simulink library "RobotControlLib"  (R2016b)
settings: Solver=VariableStepAuto  StartTime=0.0  StopTime=10.0  RelTol=1e-3
values from neighbouring files (symbols this model uses):
  CAL_EAST = int16(0)    [ControlInit.m]
  CAL_hitBackwardDist_mm = single(150)    [ControlInit.m]
  CAL_NORTH = int16(270)    [ControlInit.m]
  CAL_PwmMoveThd_mm = uint8(180)    [ControlInit.m]
  CAL_SOUTH = int16(90)    [ControlInit.m]
  CAL_WEST = int16(180)    [ControlInit.m]
  CONST_Zero = int16(0)    [ControlInit.m]
  ENU_DIAG = uint8(28)    [ControlInit.m]
  ENU_END = uint8(27)    [ControlInit.m]
  ENU_SHIFT_HEADING = uint8(29)    [ControlInit.m]
libraries: COMH x1, DSCA x1, ROTH x1, MOVH x1, SCAN x1, MOTH x1
settings Model: Creator=oelkawok  LastModifiedBy=oelkawok

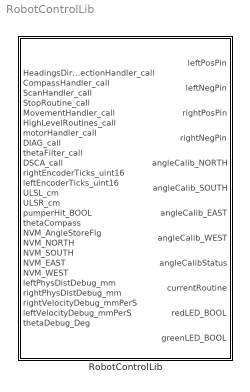
== system RobotControlLib ==
  RobotControlLib : Subsystem

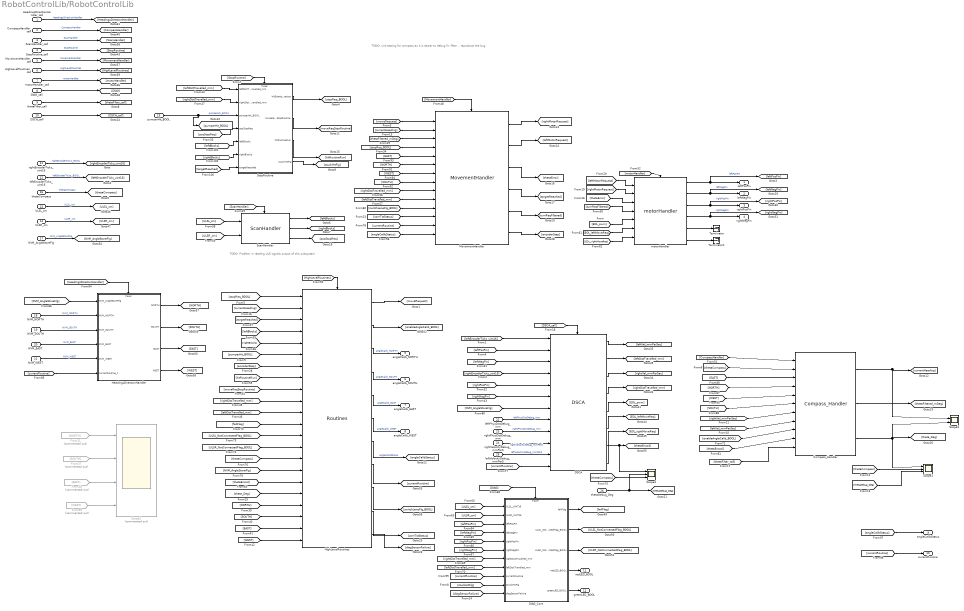
== system RobotControlLib/RobotControlLib ==
  note: TODO: Problem in reading ULS signals output of this subsystem
  note: TODO: unit testing for compass as it is easier to debug fix filter... reproduce the bug
  HeadingsDirectionHandler_call : Inport  PortDimensions=1
  CompassHandler_call : Inport  Port=2  PortDimensions=1
  ScanHandler_call : Inport  Port=3  PortDimensions=1
  StopRoutine_call : Inport  Port=4  PortDimensions=1
  MovementHandler_call : Inport  Port=5  PortDimensions=1
  HighLevelRoutines_call : Inport  Port=6  PortDimensions=1
  motorHandler_call : Inport  Port=7  PortDimensions=1
  DIAG_call : Inport  Port=8  PortDimensions=1
  thetaFilter_call : Inport  Port=9  PortDimensions=1
  DSCA_call : Inport  Port=10  PortDimensions=1
  rightEncoderTicks_uint16 : Inport  Port=11  PortDimensions=1
  leftEncoderTicks_uint16 : Inport  Port=12  PortDimensions=1
  ULSL_cm : Inport  Port=13  PortDimensions=1
  ULSR_cm : Inport  Port=14  PortDimensions=1
  pumperHit_BOOL : Inport  Port=15  OutDataTypeStr=boolean  PortDimensions=1
  thetaCompass : Inport  Port=16  OutDataTypeStr=int16  PortDimensions=1
  NVM_AngleStoreFlg : Inport  Port=17  PortDimensions=1
  NVM_NORTH : Inport  Port=18  PortDimensions=1
  NVM_SOUTH : Inport  Port=19  PortDimensions=1
  NVM_EAST : Inport  Port=20  PortDimensions=1
  NVM_WEST : Inport  Port=21  PortDimensions=1
  leftPhysDistDebug_mm : Inport  Port=22
  rightPhysDistDebug_mm : Inport  Port=23
  rightVelocityDebug_mmPerS : Inport  Port=24
  leftVelocityDebug_mmPerS : Inport  Port=25
  thetaDebug_Deg : Inport  Port=26
  Compass_Handler : COMH/Compass_Handler
  DIAG_Cont : Subsystem
      settings: RTWSystemCode=Nonreusable function  RTWFcnNameOpts=Use subsystem name  RTWFileNameOpts=Use subsystem name  FunctionInterfaceSpec=Allow arguments
  DSCA : DSCA/DSCA
  From21 : From  Commented=on  GotoTag=NORTH
  From37 : From  Commented=on  GotoTag=SOUTH
  From38 : From  Commented=on  GotoTag=EAST
  From95 : From  Commented=on  GotoTag=WEST
  HeadingsDirectionHandler : Subsystem
      settings: RTWSystemCode=Nonreusable function  RTWFcnNameOpts=Use subsystem name  RTWFileNameOpts=Use subsystem name  FunctionInterfaceSpec=Allow arguments
  HighLevelRoutines : ROTH/Routines
  MovementHandler : MOVH/MovementHandler
  ScanHandler : SCAN/ScanHandler
  Scope1 : Scope  NumInputPorts=3
  Scope2 : Scope  Commented=on  NumInputPorts=4
  Scope3 : Scope  NumInputPorts=2
  Scope4 : Scope  NumInputPorts=3
  StopRoutine : Subsystem
      settings: RTWSystemCode=Nonreusable function  RTWFcnNameOpts=Use subsystem name  RTWFileNameOpts=Use subsystem name  FunctionInterfaceSpec=Allow arguments
  Terminator : Terminator
  Terminator1 : Terminator
  motorHandler : MOTH/motorHandler
  leftPosPin : Outport  OutDataTypeStr=uint8  PortDimensions=1
      settings: AttributesFormatString=|
      | Mode: %<OutputWhenDisabled>
      | Init: %<InitialOutput>
  leftNegPin : Outport  Port=2  OutDataTypeStr=uint8  PortDimensions=1
      settings: AttributesFormatString=|
      | Mode: %<OutputWhenDisabled>
      | Init: %<InitialOutput>
  rightPosPin : Outport  Port=3  OutDataTypeStr=uint8  PortDimensions=1
      settings: AttributesFormatString=|
      | Mode: %<OutputWhenDisabled>
      | Init: %<InitialOutput>
  rightNegPin : Outport  Port=4  OutDataTypeStr=uint8  PortDimensions=1
      settings: AttributesFormatString=|
      | Mode: %<OutputWhenDisabled>
      | Init: %<InitialOutput>
  angleCalib_NORTH : Outport  Port=5  InitialOutput=0
      settings: AttributesFormatString=|
      | Mode: %<OutputWhenDisabled>
      | Init: %<InitialOutput>
  angleCalib_SOUTH : Outport  Port=6  InitialOutput=0
      settings: AttributesFormatString=|
      | Mode: %<OutputWhenDisabled>
      | Init: %<InitialOutput>
  angleCalib_EAST : Outport  Port=7  InitialOutput=0
      settings: AttributesFormatString=|
      | Mode: %<OutputWhenDisabled>
      | Init: %<InitialOutput>
  angleCalib_WEST : Outport  Port=8  InitialOutput=0
      settings: AttributesFormatString=|
      | Mode: %<OutputWhenDisabled>
      | Init: %<InitialOutput>
  angleCalibStatus : Outport  Port=9
      settings: AttributesFormatString=|
      | Mode: %<OutputWhenDisabled>
      | Init: %<InitialOutput>
  currentRoutine : Outport  Port=10
      settings: AttributesFormatString=|
      | Mode: %<OutputWhenDisabled>
      | Init: %<InitialOutput>
  redLED_BOOL : Outport  Port=11
      settings: AttributesFormatString=|
      | Mode: %<OutputWhenDisabled>
      | Init: %<InitialOutput>
  greenLED_BOOL : Outport  Port=12
      settings: AttributesFormatString=|
      | Mode: %<OutputWhenDisabled>
      | Init: %<InitialOutput>
  wires:
  [diagSensorFailure] -> DIAG_Cont/11(diagSensorFailure)
  [stuckHitFlg] -> DIAG_Cont/10(stuckHitFlg)
  HighLevelRoutines/11 -> [diagSensorFailure]
  StopRoutine/4(stuckHitFlg) -> [stuckHitFlg]
  [rightBlocks] -> StopRoutine/6(rightBlocks)
  [leftBlocks] -> StopRoutine/5(leftBlocks)
  [targetReached] -> StopRoutine/7(targetReached)
  [currentRoutine] -> DIAG_Cont/9(currentRoutine)
  DIAG_Cont/4(redLED_BOOL) -> redLED_BOOL/1
  DIAG_Cont/5(greenLED_BOOL) -> greenLED_BOOL/1
  [currentRoutine] -> currentRoutine/1
  [angleCalibStatus] -> MovementHandler/14
  [angleCalibStatus] -> angleCalibStatus/1
  From95/1 -> Scope2/4
  From38/1 -> Scope2/3
  From37/1 -> Scope2/2
  From21/1 -> Scope2/1
  [thetaDebug_Deg] -> Scope1/3
  thetaDebug_Deg/1 -> Scope4/2, [thetaDebug_Deg]
  [SOUTH] -> HighLevelRoutines/20
  [WEST] -> HighLevelRoutines/22
  [EAST] -> HighLevelRoutines/21
  [NORTH] -> HighLevelRoutines/19
  [currentRoutine] -> MovementHandler/13
  [HeadingsDirectionHandler] -> HeadingsDirectionHandler/Trigger
  HeadingsDirectionHandler_call/1 -> [HeadingsDirectionHandler]  "HeadingsDirectionHandler"
  HeadingsDirectionHandler/1(NORTH) -> [NORTH]
  HeadingsDirectionHandler/2(SOUTH) -> [SOUTH]
  HeadingsDirectionHandler/3(EAST) -> [EAST]
  HeadingsDirectionHandler/4(WEST) -> [WEST]
  [NVM_AngleStoreFlg] -> HeadingsDirectionHandler/1(NVM_AngleStoreFlg)
  [theta_Deg] -> HighLevelRoutines/18
  [comTstStatus] -> MovementHandler/12
  HighLevelRoutines/10 -> [comTstStatus]
  DIAG_call/1 -> [DIAG]
  [enableAngleCalib_BOOL] -> Compass_Handler/9
  Compass_Handler/3 -> Scope1/1, [theta_Deg], Scope3/2
  [thetaCompass] -> Scope1/2
  [switchLaneFlg_BOOL] -> MovementHandler/11
  HighLevelRoutines/9 -> [switchLaneFlg_BOOL]
  HighLevelRoutines/8 -> [currentRoutine]
  [currentRoutine] -> DSCA/12
  leftVelocityDebug_mmPerS/1 -> DSCA/11  "leftVelocityDebug_mmPerS"
  rightVelocityDebug_mmPerS/1 -> DSCA/10  "rightVelocityDebug_mmPerS"
  rightPhysDistDebug_mm/1 -> DSCA/9  "rightPhysDistDebug_mm"
  leftPhysDistDebug_mm/1 -> DSCA/8  "leftPhysDistDebug_mm"
  [thetaCompass] -> Scope4/3
  DSCA/8 -> [thetaEncod], Scope4/1
  [NVM_AngleStoreFlg] -> DSCA/7
  [NVM_AngleStoreFlg] -> HighLevelRoutines/16
  NVM_AngleStoreFlg/1 -> [NVM_AngleStoreFlg]  "NVM_AngleStoreFlg"
  HighLevelRoutines/7 -> [angleCalibStatus]  "angleCalibStatus"
  HighLevelRoutines/3 -> angleCalib_NORTH/1  "angleCalib_NORTH"
  HighLevelRoutines/4 -> angleCalib_SOUTH/1  "angleCalib_SOUTH"
  HighLevelRoutines/5 -> angleCalib_EAST/1  "angleCalib_EAST"
  HighLevelRoutines/6 -> angleCalib_WEST/1  "angleCalib_WEST"
  NVM_WEST/1 -> HeadingsDirectionHandler/5(NVM_WEST)  "NVM_WEST"
  NVM_EAST/1 -> HeadingsDirectionHandler/4(NVM_EAST)  "NVM_EAST"
  NVM_SOUTH/1 -> HeadingsDirectionHandler/3(NVM_SOUTH)  "NVM_SOUTH"
  NVM_NORTH/1 -> HeadingsDirectionHandler/2(NVM_NORTH)  "NVM_NORTH"
  [thetaCompass] -> HighLevelRoutines/15
  [thetaEncod] -> Compass_Handler/10
  HighLevelRoutines/2 -> [enableAngleCalib_BOOL]
  [ULSR_NotConnectedFlag_BOOL] -> HighLevelRoutines/14
  [ULSL_NotConnectedFlag_BOOL] -> HighLevelRoutines/13
  [failFlag] -> HighLevelRoutines/12
  DIAG_Cont/3(ULSR_NotConnectedFlag_BOOL) -> [ULSR_NotConnectedFlag_BOOL]
  DIAG_Cont/2(ULSL_NotConnectedFlag_BOOL) -> [ULSL_NotConnectedFlag_BOOL]
  DIAG_Cont/1(failFlag) -> [failFlag]
  [leftDistTravelled_mm] -> DIAG_Cont/8(leftDistTravelled_mm)
  [rightDistTravelled_mm] -> DIAG_Cont/7(rightDistTravelled_mm)
  [DIAG] -> DIAG_Cont/Trigger
  [rightNegPin] -> DIAG_Cont/6(rightNegPin)
  [rightPosPin] -> DIAG_Cont/5(rightPosPin)
  [leftNegPin] -> DIAG_Cont/4(leftNegPin)
  [leftPosPin] -> DIAG_Cont/3(leftPosPin)
  [ULSL_cm] -> DIAG_Cont/1(ULSL_UINT16)
  [ULSR_cm] -> DIAG_Cont/2(ULSR_UINT16)
  [ULSR_cm] -> ScanHandler/2
  [ULSL_cm] -> ScanHandler/1
  ULSR_cm/1 -> [ULSR_cm]  "ULSR_cm"
  ULSL_cm/1 -> [ULSL_cm]  "ULSL_cm"
  DSCA/7 -> [EOL_rightMoveReq]
  DSCA/6 -> [EOL_leftMoveReq]
  DSCA/5 -> [EOL_pwm]
  [EOL_pwm] -> motorHandler/5
  [EOL_leftMoveReq] -> motorHandler/6
  [EOL_rightMoveReq] -> motorHandler/7
  [leftDistTravelled_mm] -> MovementHandler/10
  [leftDistTravelled_mm] -> HighLevelRoutines/11
  [rightDistTravelled_mm] -> HighLevelRoutines/10
  [rightDistTravelled_mm] -> MovementHandler/9
  motorHandler_call/1 -> [motorHandler]  "motorHandler"
  CompassHandler_call/1 -> [CompassHandler]  "CompassHandler"
  HighLevelRoutines_call/1 -> [HighLevelRoutines]  "HighLevelRoutines"
  ScanHandler_call/1 -> [ScanHandler]  "ScanHandler"
  StopRoutine_call/1 -> [StopRoutine]  "StopRoutine"
  MovementHandler_call/1 -> [MovementHandler]  "MovementHandler"
  [moveReqStopRoutine] -> HighLevelRoutines/9
  [hitRoutineRun] -> HighLevelRoutines/8
  HighLevelRoutines/1 -> [moveRequest]
  [thetaFiltered_mDeg] -> MovementHandler/3
  [currentHeading] -> MovementHandler/2
  ScanHandler/3 -> [posStopReq]
  [moveRequest] -> MovementHandler/1
  [stopReq_BOOL] -> MovementHandler/4
  [SOUTH] -> MovementHandler/8
  [WEST] -> MovementHandler/7
  [NORTH] -> MovementHandler/6
  [EAST] -> MovementHandler/5
  [SOUTH] -> Compass_Handler/6
  [WEST] -> Compass_Handler/5
  [NORTH] -> Compass_Handler/4
  [EAST] -> Compass_Handler/3
  [stopReq_BOOL] -> HighLevelRoutines/1
  [currentHeading] -> HighLevelRoutines/2
  [encoderStep] -> HighLevelRoutines/7
  StopRoutine/1(hitEvents_vector) -> [stopReq_BOOL]
  Compass_Handler/2 -> [thetaFiltered_mDeg]
  [pumperHit_BOOL] -> HighLevelRoutines/6
  StopRoutine/2(moveReqStopRoutine) -> [moveReqStopRoutine]
  StopRoutine/3(hitRoutineRun) -> [hitRoutineRun]
  MovementHandler/6 -> [encoderStep]
  [rightVel_mmPerSec] -> Compass_Handler/7
  [leftVel_mmPerSec] -> Compass_Handler/8
  motorHandler/6 -> Terminator1/1
  motorHandler/5 -> Terminator/1
  pumperHit_BOOL/1 -> StopRoutine/3(pumperHit_BOOL), [pumperHit_BOOL]  "pumperHit_BOOL"
  thetaCompass/1 -> [thetaCompass]  "thetaCompass"
  MovementHandler/5 -> [turnReqFiltered]
  [turnReqFiltered] -> motorHandler/4
  [targetReached] -> HighLevelRoutines/3
  [posStopReq] -> StopRoutine/4(posStopReq)
  [rightBlocks] -> HighLevelRoutines/5
  [leftBlocks] -> HighLevelRoutines/4
  motorHandler/4 -> [rightNegPin], rightNegPin/1  "rightNegPin"
  motorHandler/2 -> [leftNegPin], leftNegPin/1  "leftNegPin"
  motorHandler/3 -> [rightPosPin], rightPosPin/1  "rightPosPin"
  motorHandler/1 -> [leftPosPin], leftPosPin/1  "leftPosPin"
  MovementHandler/3 -> [thetaError]
  [thetaError] -> motorHandler/3
  MovementHandler/4 -> [targetReached]
  rightEncoderTicks_uint16/1 -> [rightEncoderTicks_uint16]  "rightEncoderTicks_BOOL"
  ScanHandler/2 -> [rightBlocks]
  [thetaCompass] -> Compass_Handler/2
  ScanHandler/1 -> [leftBlocks]
  Compass_Handler/1 -> [currentHeading], Scope3/1
  [rightMotorRequest] -> motorHandler/2
  [leftMotorRequest] -> motorHandler/1
  MovementHandler/2 -> [leftMotorRequest]
  MovementHandler/1 -> [rightMotorRequest]
  leftEncoderTicks_uint16/1 -> [leftEncoderTicks_uint16]  "leftEncoderTicks_BOOL"
  [leftEncoderTicks_uint16] -> DSCA/1
  [rightEncoderTicks_uint16] -> DSCA/4
  DSCA/2 -> [leftDistTravelled_mm]
  DSCA/3 -> [rightVel_mmPerSec]
  DSCA/4 -> [rightDistTravelled_mm]
  DSCA/1 -> [leftVel_mmPerSec]
  [rightDistTravelled_mm] -> StopRoutine/2(rightDistTravelled_mm)
  [leftDistTravelled_mm] -> StopRoutine/1(leftDistTravelled_mm)
  [StopRoutine] -> StopRoutine/Trigger
  [MovementHandler] -> MovementHandler/Trigger
  [ScanHandler] -> ScanHandler/Trigger
  [motorHandler] -> motorHandler/Trigger
  [CompassHandler] -> Compass_Handler/1
  [HighLevelRoutines] -> HighLevelRoutines/Trigger
  [leftPosPin] -> DSCA/2
  [leftNegPin] -> DSCA/3
  [rightPosPin] -> DSCA/5
  [rightNegPin] -> DSCA/6
  [thetaEncod] -> HighLevelRoutines/17
  [currentRoutine] -> HeadingsDirectionHandler/6(currentRoutine_z)
  thetaFilter_call/1 -> [thetaFilter_call]
  DSCA_call/1 -> [DSCA_call]
  [DSCA_call] -> DSCA/Trigger
  [thetaFilter_call] -> Compass_Handler/11

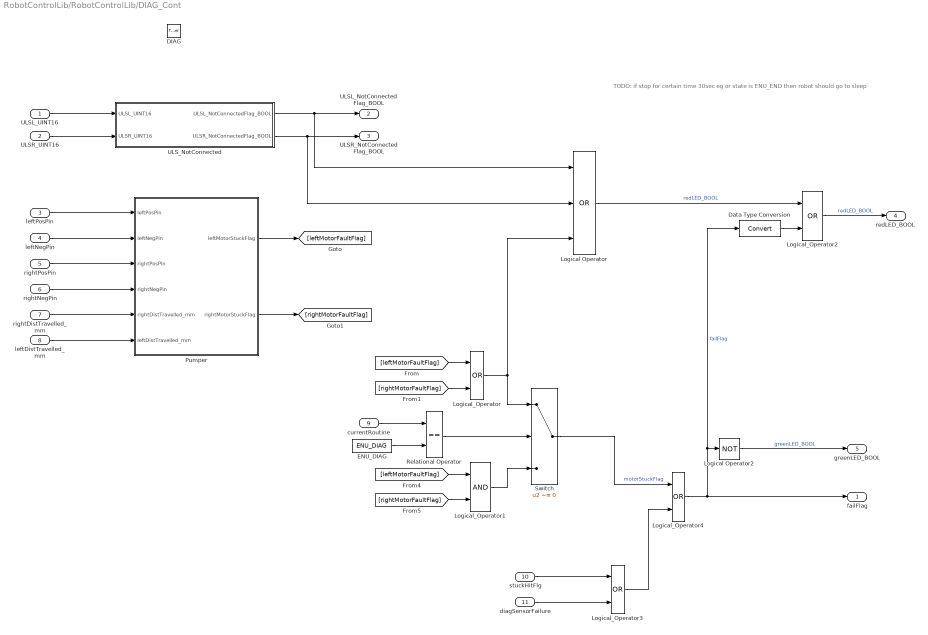
== system RobotControlLib/RobotControlLib/DIAG_Cont ==
  note: TODO: if stop for certain time 30sec eg or state is ENU_END then robot should go to sleep
  ULSL_UINT16 : Inport  PortDimensions=1
  ULSR_UINT16 : Inport  Port=2  PortDimensions=1
  leftPosPin : Inport  Port=3  PortDimensions=1
  leftNegPin : Inport  Port=4  PortDimensions=1
  rightPosPin : Inport  Port=5  PortDimensions=1
  rightNegPin : Inport  Port=6  PortDimensions=1
  rightDistTravelled_mm : Inport  Port=7  PortDimensions=1
  leftDistTravelled_mm : Inport  Port=8  PortDimensions=1
  currentRoutine : Inport  Port=9  PortDimensions=1
  stuckHitFlg : Inport  Port=10  PortDimensions=1
  diagSensorFailure : Inport  Port=11  PortDimensions=1
  DIAG : TriggerPort  TriggerType=function-call  VariantControl=Variant
      settings: AttributesFormatString=Mode: %<StatesWhenEnabling>
  Data Type Conversion : DataTypeConversion
  ENU_DIAG : Constant  Value=ENU_DIAG
  Logical Operator : Logic  Operator=OR  Inputs=3  AllPortsSameDT=off  OutDataTypeStr=boolean
  Logical Operator2 : Logic  Operator=NOT  IconShape=distinctive  AllPortsSameDT=off  OutDataTypeStr=boolean
  Logical_Operator{,2..4} (4 alike) : Logic  Operator=OR  AllPortsSameDT=off  OutDataTypeStr=boolean
  Logical_Operator1 : Logic  AllPortsSameDT=off  OutDataTypeStr=boolean
  Pumper : Subsystem
  Relational Operator : RelationalOperator  Operator===  OutDataTypeStr=boolean  RndMeth=Simplest
  Switch : Switch  Criteria=u2 ~= 0
  ULS_NotConnected : Subsystem
  failFlag : Outport
      settings: AttributesFormatString=|
      | Mode: %<OutputWhenDisabled>
      | Init: %<InitialOutput>
  ULSL_NotConnectedFlag_BOOL : Outport  Port=2
      settings: AttributesFormatString=|
      | Mode: %<OutputWhenDisabled>
      | Init: %<InitialOutput>
  ULSR_NotConnectedFlag_BOOL : Outport  Port=3
      settings: AttributesFormatString=|
      | Mode: %<OutputWhenDisabled>
      | Init: %<InitialOutput>
  redLED_BOOL : Outport  Port=4
  greenLED_BOOL : Outport  Port=5
  wires:
  Data Type Conversion/1 -> Logical_Operator2/2
  Logical_Operator4/1 -> failFlag/1, Logical Operator2/1, Data Type Conversion/1  "failFlag"
  Logical_Operator3/1 -> Logical_Operator4/2
  diagSensorFailure/1 -> Logical_Operator3/2
  stuckHitFlg/1 -> Logical_Operator3/1
  Logical Operator/1 -> Logical_Operator2/1  "redLED_BOOL"
  Logical_Operator1/1 -> Switch/3
  [rightMotorFaultFlag] -> Logical_Operator1/2
  [leftMotorFaultFlag] -> Logical_Operator1/1
  Logical_Operator/1 -> Logical Operator/3, Switch/1
  Relational Operator/1 -> Switch/2
  ENU_DIAG/1 -> Relational Operator/2
  currentRoutine/1 -> Relational Operator/1
  [rightMotorFaultFlag] -> Logical_Operator/2
  [leftMotorFaultFlag] -> Logical_Operator/1
  Logical Operator2/1 -> greenLED_BOOL/1  "greenLED_BOOL"
  Logical_Operator2/1 -> redLED_BOOL/1  "redLED_BOOL"
  rightDistTravelled_mm/1 -> Pumper/5(rightDistTravelled_mm)
  ULS_NotConnected/2(ULSR_NotConnectedFlag_BOOL) -> ULSR_NotConnectedFlag_BOOL/1, Logical Operator/2
  ULS_NotConnected/1(ULSL_NotConnectedFlag_BOOL) -> ULSL_NotConnectedFlag_BOOL/1, Logical Operator/1
  Switch/1 -> Logical_Operator4/1  "motorStuckFlag"
  Pumper/2(rightMotorStuckFlag) -> [rightMotorFaultFlag]
  Pumper/1(leftMotorStuckFlag) -> [leftMotorFaultFlag]
  leftDistTravelled_mm/1 -> Pumper/6(leftDistTravelled_mm)
  rightNegPin/1 -> Pumper/4(rightNegPin)
  leftPosPin/1 -> Pumper/1(leftPosPin)
  rightPosPin/1 -> Pumper/3(rightPosPin)
  leftNegPin/1 -> Pumper/2(leftNegPin)
  ULSR_UINT16/1 -> ULS_NotConnected/2(ULSR_UINT16)
  ULSL_UINT16/1 -> ULS_NotConnected/1(ULSL_UINT16)

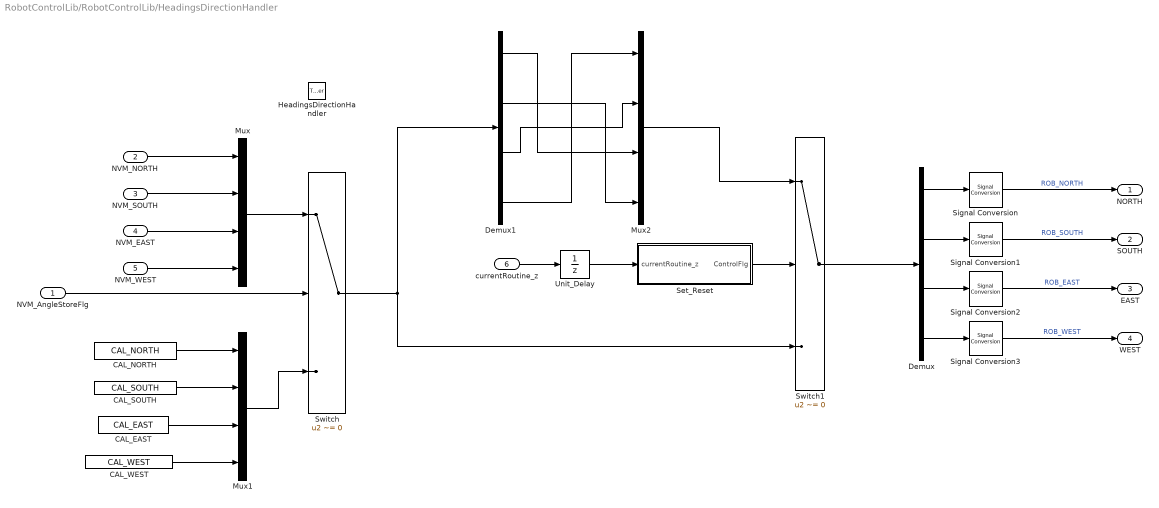
== system RobotControlLib/RobotControlLib/HeadingsDirectionHandler ==
  NVM_AngleStoreFlg : Inport  PortDimensions=1
  NVM_NORTH : Inport  Port=2  PortDimensions=1
  NVM_SOUTH : Inport  Port=3  PortDimensions=1
  NVM_EAST : Inport  Port=4  PortDimensions=1
  NVM_WEST : Inport  Port=5  PortDimensions=1
  currentRoutine_z : Inport  Port=6  PortDimensions=1
  HeadingsDirectionHandler : TriggerPort  TriggerType=function-call  VariantControl=Variant
      settings: AttributesFormatString=Mode: %<StatesWhenEnabling>
  CAL_EAST : Constant  Value=CAL_EAST
  CAL_NORTH : Constant  Value=CAL_NORTH
  CAL_SOUTH : Constant  Value=CAL_SOUTH
  CAL_WEST : Constant  Value=CAL_WEST
  Demux : Demux
  Demux1 : Demux
  Mux : Mux
  Mux1 : Mux
  Mux2 : Mux
  Set_Reset : Subsystem
  Signal Conversion{,1..3} (4 alike) : SignalConversion  OverrideOpt=off
  Switch : Switch  Criteria=u2 ~= 0
  Switch1 : Switch  Criteria=u2 ~= 0
  Unit_Delay : UnitDelay  InitialCondition=ENU_END  SampleTime=-1
      settings: AttributesFormatString=Init: %<InitialCondition>
  NORTH : Outport
  SOUTH : Outport  Port=2
  EAST : Outport  Port=3
  WEST : Outport  Port=4
  wires:
  Set_Reset/1(ControlFlg) -> Switch1/2
  Mux2/1 -> Switch1/1
  Switch/1 -> Demux1/1, Switch1/3
  Switch1/1 -> Demux/1
  Demux1/3 -> Mux2/2
  Demux1/2 -> Mux2/4
  Demux1/1 -> Mux2/3
  Demux1/4 -> Mux2/1
  NVM_WEST/1 -> Mux/4
  NVM_EAST/1 -> Mux/3
  NVM_SOUTH/1 -> Mux/2
  NVM_NORTH/1 -> Mux/1
  Mux/1 -> Switch/1
  CAL_NORTH/1 -> Mux1/1
  CAL_SOUTH/1 -> Mux1/2
  CAL_WEST/1 -> Mux1/4
  CAL_EAST/1 -> Mux1/3
  Mux1/1 -> Switch/3
  NVM_AngleStoreFlg/1 -> Switch/2
  Signal Conversion1/1 -> SOUTH/1  "ROB_SOUTH"
  Demux/1 -> Signal Conversion/1
  Signal Conversion2/1 -> EAST/1  "ROB_EAST"
  Signal Conversion3/1 -> WEST/1  "ROB_WEST"
  Unit_Delay/1 -> Set_Reset/1(currentRoutine_z)
  currentRoutine_z/1 -> Unit_Delay/1
  Signal Conversion/1 -> NORTH/1  "ROB_NORTH"
  Demux/2 -> Signal Conversion1/1
  Demux/3 -> Signal Conversion2/1
  Demux/4 -> Signal Conversion3/1

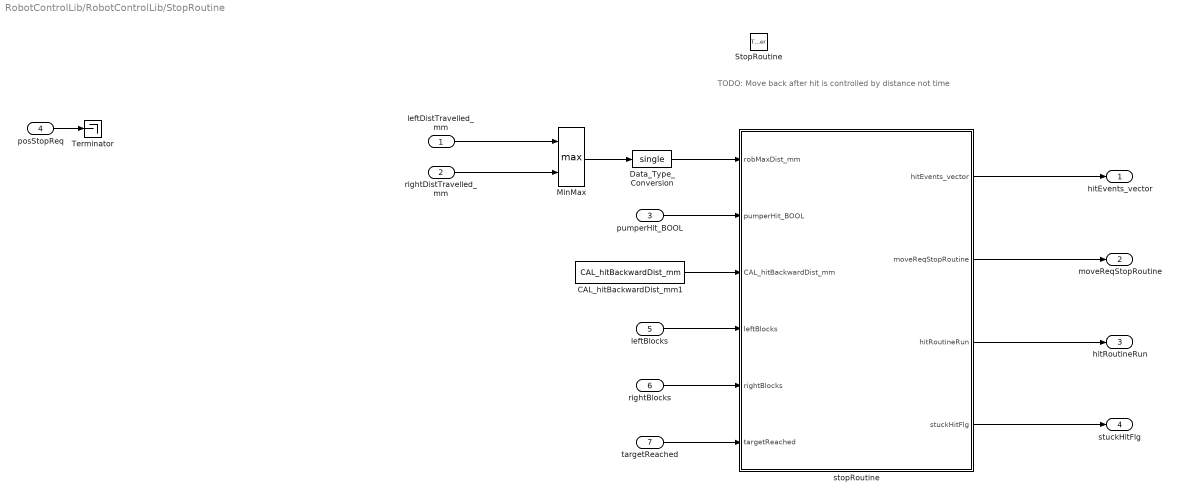
== system RobotControlLib/RobotControlLib/StopRoutine ==
  note: TODO: Move back after hit is controlled by distance not time
  leftDistTravelled_mm : Inport
  rightDistTravelled_mm : Inport  Port=2
  pumperHit_BOOL : Inport  Port=3
  posStopReq : Inport  Port=4
  leftBlocks : Inport  Port=5
  rightBlocks : Inport  Port=6
  targetReached : Inport  Port=7
  StopRoutine : TriggerPort  TriggerType=function-call  VariantControl=Variant
      settings: AttributesFormatString=Mode: %<StatesWhenEnabling>
  CAL_hitBackwardDist_mm1 : Constant  Value=CAL_hitBackwardDist_mm
  Data_Type_Conversion : DataTypeConversion  OutDataTypeStr=single
  MinMax : MinMax  Function=max  Inputs=2
  Terminator : Terminator
  stopRoutine : Subsystem
  hitEvents_vector : Outport
      settings: AttributesFormatString=|
      | Mode: %<OutputWhenDisabled>
      | Init: %<InitialOutput>
  moveReqStopRoutine : Outport  Port=2
      settings: AttributesFormatString=|
      | Mode: %<OutputWhenDisabled>
      | Init: %<InitialOutput>
  hitRoutineRun : Outport  Port=3
      settings: AttributesFormatString=|
      | Mode: %<OutputWhenDisabled>
      | Init: %<InitialOutput>
  stuckHitFlg : Outport  Port=4
      settings: AttributesFormatString=|
      | Mode: %<OutputWhenDisabled>
      | Init: %<InitialOutput>
  wires:
  stopRoutine/4(stuckHitFlg) -> stuckHitFlg/1
  targetReached/1 -> stopRoutine/6(targetReached)
  rightBlocks/1 -> stopRoutine/5(rightBlocks)
  leftBlocks/1 -> stopRoutine/4(leftBlocks)
  stopRoutine/3(hitRoutineRun) -> hitRoutineRun/1
  stopRoutine/2(moveReqStopRoutine) -> moveReqStopRoutine/1
  stopRoutine/1(hitEvents_vector) -> hitEvents_vector/1
  CAL_hitBackwardDist_mm1/1 -> stopRoutine/3(CAL_hitBackwardDist_mm)
  Data_Type_Conversion/1 -> stopRoutine/1(robMaxDist_mm)
  posStopReq/1 -> Terminator/1
  pumperHit_BOOL/1 -> stopRoutine/2(pumperHit_BOOL)
  leftDistTravelled_mm/1 -> MinMax/1
  rightDistTravelled_mm/1 -> MinMax/2
  MinMax/1 -> Data_Type_Conversion/1

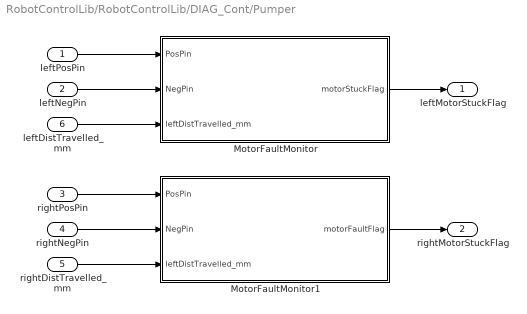
== system RobotControlLib/RobotControlLib/DIAG_Cont/Pumper ==
  leftPosPin : Inport  PortDimensions=1
  leftNegPin : Inport  Port=2  PortDimensions=1
  rightPosPin : Inport  Port=3  PortDimensions=1
  rightNegPin : Inport  Port=4  PortDimensions=1
  rightDistTravelled_mm : Inport  Port=5  PortDimensions=1
  leftDistTravelled_mm : Inport  Port=6  PortDimensions=1
  MotorFaultMonitor : Subsystem
  MotorFaultMonitor1 : Subsystem
  leftMotorStuckFlag : Outport
  rightMotorStuckFlag : Outport  Port=2
  wires:
  MotorFaultMonitor1/1(motorFaultFlag) -> rightMotorStuckFlag/1
  rightPosPin/1 -> MotorFaultMonitor1/1(PosPin)
  rightNegPin/1 -> MotorFaultMonitor1/2(NegPin)
  rightDistTravelled_mm/1 -> MotorFaultMonitor1/3(leftDistTravelled_mm)
  MotorFaultMonitor/1(motorStuckFlag) -> leftMotorStuckFlag/1
  leftDistTravelled_mm/1 -> MotorFaultMonitor/3(leftDistTravelled_mm)
  leftNegPin/1 -> MotorFaultMonitor/2(NegPin)
  leftPosPin/1 -> MotorFaultMonitor/1(PosPin)

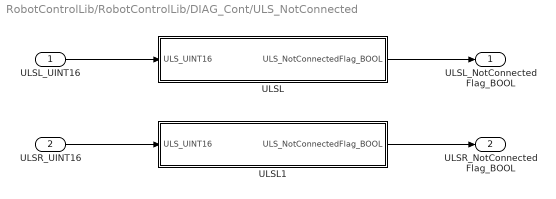
== system RobotControlLib/RobotControlLib/DIAG_Cont/ULS_NotConnected ==
  ULSL_UINT16 : Inport  PortDimensions=1
  ULSR_UINT16 : Inport  Port=2  PortDimensions=1
  ULSL : Subsystem
  ULSL1 : Subsystem
  ULSL_NotConnectedFlag_BOOL : Outport
  ULSR_NotConnectedFlag_BOOL : Outport  Port=2
  wires:
  ULSL1/1(ULS_NotConnectedFlag_BOOL) -> ULSR_NotConnectedFlag_BOOL/1
  ULSL/1(ULS_NotConnectedFlag_BOOL) -> ULSL_NotConnectedFlag_BOOL/1
  ULSR_UINT16/1 -> ULSL1/1(ULS_UINT16)
  ULSL_UINT16/1 -> ULSL/1(ULS_UINT16)

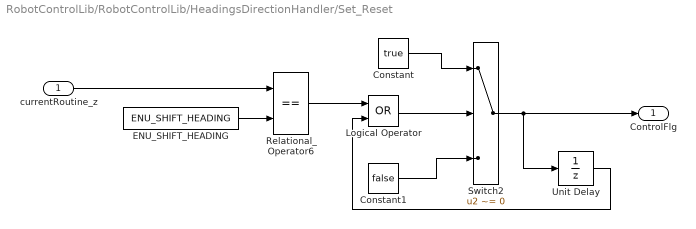
== system RobotControlLib/RobotControlLib/HeadingsDirectionHandler/Set_Reset ==
  currentRoutine_z : Inport  PortDimensions=1
  Constant : Constant  Value=true
  Constant1 : Constant  Value=false
  ENU_SHIFT_HEADING : Constant  Value=ENU_SHIFT_HEADING
  Logical Operator : Logic  Operator=OR  AllPortsSameDT=off  OutDataTypeStr=boolean
  Relational_Operator6 : RelationalOperator  Operator===  OutDataTypeStr=boolean  RndMeth=Nearest
  Switch2 : Switch  Criteria=u2 ~= 0
  Unit Delay : UnitDelay  SampleTime=-1
  ControlFlg : Outport
  wires:
  Relational_Operator6/1 -> Logical Operator/1
  currentRoutine_z/1 -> Relational_Operator6/1
  Logical Operator/1 -> Switch2/2
  Constant/1 -> Switch2/1
  Switch2/1 -> Unit Delay/1, ControlFlg/1
  Constant1/1 -> Switch2/3
  Unit Delay/1 -> Logical Operator/2
  ENU_SHIFT_HEADING/1 -> Relational_Operator6/2

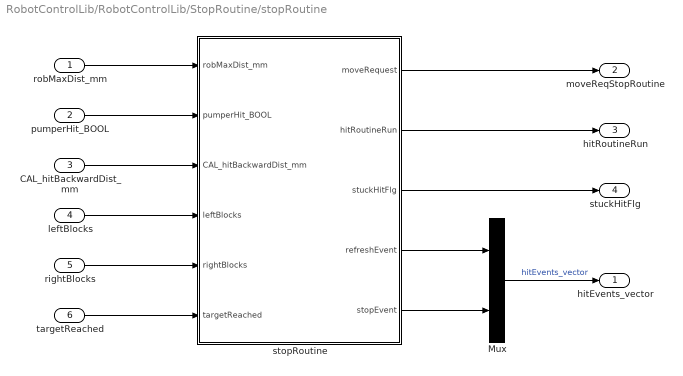
== system RobotControlLib/RobotControlLib/StopRoutine/stopRoutine ==
  robMaxDist_mm : Inport
  pumperHit_BOOL : Inport  Port=2
  CAL_hitBackwardDist_mm : Inport  Port=3
  leftBlocks : Inport  Port=4
  rightBlocks : Inport  Port=5
  targetReached : Inport  Port=6
  Mux : Mux  Inputs=2
  stopRoutine : Stateflow chart  TreatAsAtomicUnit=on
  hitEvents_vector : Outport
      settings: AttributesFormatString=|
      | Mode: %<OutputWhenDisabled>
      | Init: %<InitialOutput>
  moveReqStopRoutine : Outport  Port=2
      settings: AttributesFormatString=|
      | Mode: %<OutputWhenDisabled>
      | Init: %<InitialOutput>
  hitRoutineRun : Outport  Port=3
      settings: AttributesFormatString=|
      | Mode: %<OutputWhenDisabled>
      | Init: %<InitialOutput>
  stuckHitFlg : Outport  Port=4
      settings: AttributesFormatString=|
      | Mode: %<OutputWhenDisabled>
      | Init: %<InitialOutput>
  wires:
  stopRoutine/3(stuckHitFlg) -> stuckHitFlg/1
  rightBlocks/1 -> stopRoutine/5(rightBlocks)
  targetReached/1 -> stopRoutine/6(targetReached)
  leftBlocks/1 -> stopRoutine/4(leftBlocks)
  pumperHit_BOOL/1 -> stopRoutine/2(pumperHit_BOOL)
  Mux/1 -> hitEvents_vector/1  "hitEvents_vector"
  stopRoutine/5(stopEvent) -> Mux/2
  stopRoutine/4(refreshEvent) -> Mux/1
  stopRoutine/2(hitRoutineRun) -> hitRoutineRun/1
  CAL_hitBackwardDist_mm/1 -> stopRoutine/3(CAL_hitBackwardDist_mm)
  robMaxDist_mm/1 -> stopRoutine/1(robMaxDist_mm)
  stopRoutine/1(moveRequest) -> moveReqStopRoutine/1

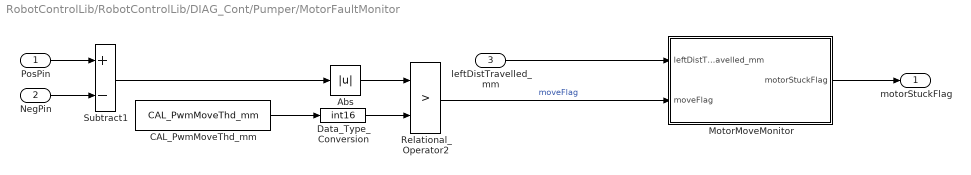
== system RobotControlLib/RobotControlLib/DIAG_Cont/Pumper/MotorFaultMonitor ==
  PosPin : Inport  PortDimensions=1
  NegPin : Inport  Port=2  PortDimensions=1
  leftDistTravelled_mm : Inport  Port=3  PortDimensions=1
  Abs : Abs  SaturateOnIntegerOverflow=on
  CAL_PwmMoveThd_mm : Constant  Value=CAL_PwmMoveThd_mm
  Data_Type_Conversion : DataTypeConversion  OutDataTypeStr=int16
  MotorMoveMonitor : Subsystem
  Relational_Operator2 : RelationalOperator  Operator=>  OutDataTypeStr=boolean  RndMeth=Simplest
  Subtract1 : Sum  Inputs=+-  OutDataTypeStr=int16
  motorStuckFlag : Outport
  wires:
  MotorMoveMonitor/1(motorStuckFlag) -> motorStuckFlag/1
  Relational_Operator2/1 -> MotorMoveMonitor/2(moveFlag)  "moveFlag"
  leftDistTravelled_mm/1 -> MotorMoveMonitor/1(leftDistTravelled_mm)
  Data_Type_Conversion/1 -> Relational_Operator2/2
  NegPin/1 -> Subtract1/2
  PosPin/1 -> Subtract1/1
  CAL_PwmMoveThd_mm/1 -> Data_Type_Conversion/1
  Subtract1/1 -> Abs/1
  Abs/1 -> Relational_Operator2/1

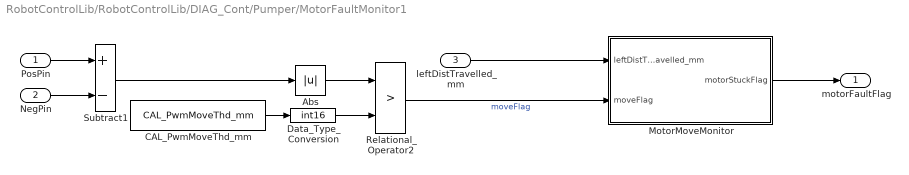
== system RobotControlLib/RobotControlLib/DIAG_Cont/Pumper/MotorFaultMonitor1 ==
  PosPin : Inport  PortDimensions=1
  NegPin : Inport  Port=2  PortDimensions=1
  leftDistTravelled_mm : Inport  Port=3  PortDimensions=1
  Abs : Abs  SaturateOnIntegerOverflow=on
  CAL_PwmMoveThd_mm : Constant  Value=CAL_PwmMoveThd_mm
  Data_Type_Conversion : DataTypeConversion  OutDataTypeStr=int16
  MotorMoveMonitor : Subsystem
  Relational_Operator2 : RelationalOperator  Operator=>  OutDataTypeStr=boolean  RndMeth=Simplest
  Subtract1 : Sum  Inputs=+-  OutDataTypeStr=int16
  motorFaultFlag : Outport
  wires:
  Data_Type_Conversion/1 -> Relational_Operator2/2
  leftDistTravelled_mm/1 -> MotorMoveMonitor/1(leftDistTravelled_mm)
  Relational_Operator2/1 -> MotorMoveMonitor/2(moveFlag)  "moveFlag"
  Abs/1 -> Relational_Operator2/1
  MotorMoveMonitor/1(motorStuckFlag) -> motorFaultFlag/1
  Subtract1/1 -> Abs/1
  CAL_PwmMoveThd_mm/1 -> Data_Type_Conversion/1
  PosPin/1 -> Subtract1/1
  NegPin/1 -> Subtract1/2

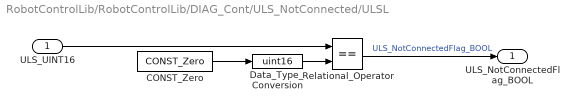
== system RobotControlLib/RobotControlLib/DIAG_Cont/ULS_NotConnected/ULSL ==
  ULS_UINT16 : Inport  PortDimensions=1
  CONST_Zero : Constant  Value=CONST_Zero
  Data_Type_Conversion : DataTypeConversion  OutDataTypeStr=uint16
  Relational_Operator : RelationalOperator  Operator===  OutDataTypeStr=boolean  RndMeth=Simplest
  ULS_NotConnectedFlag_BOOL : Outport
  wires:
  Data_Type_Conversion/1 -> Relational_Operator/2
  Relational_Operator/1 -> ULS_NotConnectedFlag_BOOL/1  "ULS_NotConnectedFlag_BOOL"
  ULS_UINT16/1 -> Relational_Operator/1
  CONST_Zero/1 -> Data_Type_Conversion/1

== system RobotControlLib/RobotControlLib/DIAG_Cont/ULS_NotConnected/ULSL1 ==
  ULS_UINT16 : Inport  PortDimensions=1
  CONST_Zero : Constant  Value=CONST_Zero
  Data_Type_Conversion : DataTypeConversion  OutDataTypeStr=uint16
  Relational_Operator : RelationalOperator  Operator===  OutDataTypeStr=boolean  RndMeth=Simplest
  ULS_NotConnectedFlag_BOOL : Outport
  wires:
  CONST_Zero/1 -> Data_Type_Conversion/1
  ULS_UINT16/1 -> Relational_Operator/1
  Relational_Operator/1 -> ULS_NotConnectedFlag_BOOL/1  "ULS_NotConnectedFlag_BOOL"
  Data_Type_Conversion/1 -> Relational_Operator/2

== system RobotControlLib/RobotControlLib/DIAG_Cont/Pumper/MotorFaultMonitor/MotorMoveMonitor ==
  leftDistTravelled_mm : Inport
  moveFlag : Inport  Port=2
  Data Type Conversion2 : DataTypeConversion
  MotorMoveMonitor : Stateflow chart  TreatAsAtomicUnit=on
  motorStuckFlag : Outport
  wires:
  Data Type Conversion2/1 -> MotorMoveMonitor/1(motorDist)
  moveFlag/1 -> MotorMoveMonitor/2(moveFlag)
  leftDistTravelled_mm/1 -> Data Type Conversion2/1
  MotorMoveMonitor/1(motorFaultFlag) -> motorStuckFlag/1

== system RobotControlLib/RobotControlLib/DIAG_Cont/Pumper/MotorFaultMonitor1/MotorMoveMonitor ==
  leftDistTravelled_mm : Inport
  moveFlag : Inport  Port=2
  Data Type Conversion2 : DataTypeConversion
  MotorMoveMonitor : Stateflow chart  TreatAsAtomicUnit=on
  motorStuckFlag : Outport
  wires:
  Data Type Conversion2/1 -> MotorMoveMonitor/1(motorDist)
  moveFlag/1 -> MotorMoveMonitor/2(moveFlag)
  leftDistTravelled_mm/1 -> Data Type Conversion2/1
  MotorMoveMonitor/1(motorFaultFlag) -> motorStuckFlag/1

== stateflow chart RobotControlLib/DIAG_Cont/Pumper/MotorFaultMonitor1/MotorMoveMonitor/MotorMoveMonitor ==
  settings: description=chart that monitor motor movement. detects if voltage is given to the mode however not encoder indication that the motor is rotating. this means motor is either stuck (high current) or encoder signal has stopped.
  state moveStart
  state moveRefresh
  state moveFault
    en:
    motorFaultFlag = true;
  (default) -> moveRefresh
  moveRefresh -> moveStart : [moveFlag]/tempDist = motorDist;
  moveStart -> (junction 6) : [after(CONST_ENCOD_TIMER_FAULT, tick) ...
      | || (moveFlag == false)]
  (junction 6) -> moveRefresh [order 2]
  (junction 6) -> moveFault [order 1] : [(moveFlag == true) &&...
      | motorDist == tempDist]
  data: tempDist local single; motorDist input; moveFlag input; motorFaultFlag output boolean; CONST_ENCOD_TIMER_FAULT constant uint8 =CONST_ENCOD_TIMER_FAULT

== stateflow chart RobotControlLib/StopRoutine/stopRoutine/stopRoutine ==
  settings: description=handles the stop routine. stop motors move backward for certain distance and proceed
  state stopRoutine
    on every(1,tick):
    send(refreshEvent);
    state CompleteStuck
      en:
      moveRequest = STOP;
      stuckHitFlg = true;
      du:
      moveRequest = STOP;
    state sideStuck
      state turnLeft
        en:
        moveRequest = ENU_MOVE_TURN_LEFT;
      state turnRight
        en:
        moveRequest = ENU_MOVE_TURN_RIGHT;
      state turnComplete
        en:
        moveRequest = FORWARD;
        hitDistance = robMaxDist_mm;
      state turnComplete1
        en:
        moveRequest = FORWARD;
        hitDistance = robMaxDist_mm;
      state GetBakRight
        en:
        moveRequest = ENU_MOVE_TURN_RIGHT;
      state GetBakLeft
        en:
        moveRequest = ENU_MOVE_TURN_LEFT;
      state escapeComplete
        en:
        moveRequest = STOP;
        escapeFlg = true;
      (default) -> (junction 34)
      (junction 34) -> turnLeft [order 2] : [leftBlocks > rightBlocks]
      (junction 34) -> turnRight [order 1] : [leftBlocks < rightBlocks]
      (junction 34) -> turnLeft [order 3]
      turnRight -> turnComplete1 : [targetReached  ...
          | && after(CONST_TARGET_REACHED_BLIND, tick)]
      turnLeft -> turnComplete : [(targetReached) ...
          | && after(CONST_TARGET_REACHED_BLIND, tick)]
      turnComplete -> GetBakRight : [((robMaxDist_mm - hitDistance)...
          |   > CAL_hitEscapeDist_mm)]
      turnComplete1 -> GetBakLeft : [((robMaxDist_mm - hitDistance)...
          |   > CAL_hitEscapeDist_mm)]
      GetBakLeft -> (junction 62)
      GetBakRight -> (junction 62)
      (junction 62) -> escapeComplete : [(targetReached) && after(5, tick)]
    state hitFinish
      en:
      moveRequest = STOP;
    state Run
    state HitStop
      en:
      moveRequest = STOP;
    state backup
      en:
      hitDistance = robMaxDist_mm;
      moveRequest = BACKWARD;
    sideStuck -> CompleteStuck [order 2] : [after(CAL_sideStuckTimeout, tick)]
        | //0.005*5000 = 25sec
    hitFinish -> sideStuck [order 2] : [after(CAL_hitBakTimeout, tick)]
        | /escapeFlg = false;
        | //0.005*400 = 2sec
    sideStuck -> Run [order 1] : [escapeFlg]
        | /hitRoutineRun = false;
        | send(stopEvent);
    (default) -> Run
    hitFinish -> Run [order 1] : [!pumperHit_BOOL]
        | /hitRoutineRun = false;
        | send(stopEvent);
    backup -> hitFinish : [((hitDistance - robMaxDist_mm)...
        |   > CAL_hitBackwardDist_mm)]
    Run -> HitStop : [pumperHit_BOOL]
        | /hitRoutineRun = true;
    HitStop -> backup : [after(CONST_CONFIRM_TIME_STOP,tick)]
  (default) -> stopRoutine
  data: robMaxDist_mm input; pumperHit_BOOL input; BACKWARD constant uint8 =ENU_BACKWARD; STOP constant uint8 =ENU_STOP; moveRequest output uint8; hitRoutineRun output boolean; CAL_hitBackwardDist_mm input =CAL_backwardTicks; hitDistance local single; CONST_CONFIRM_TIME_STOP constant uint8 =CONST_CONFIRM_TIME_STOP; leftBlocks input; rightBlocks input; targetReached input; ENU_MOVE_TURN_LEFT constant uint8 =ENU_MOVE_TURN_LEFT; ENU_MOVE_TURN_RIGHT constant uint8 =ENU_MOVE_TURN_RIGHT; FORWARD constant uint8 =ENU_FORWARD; escapeFlg local boolean; CAL_hitEscapeDist_mm constant uint16 =CAL_hitEscapeDist_mm; CAL_hitBakTimeout constant uint16 =CAL_hitBakTimeout; CAL_sideStuckTimeout constant uint16 =CAL_sideStuckTimeout; CONST_TARGET_REACHED_BLIND constant uint16 =CONST_TARGET_REACHED_BLIND; stuckHitFlg output boolean
  events: refreshEvent output EITHER_EDGE_EVENT; stopEvent output EITHER_EDGE_EVENT

== stateflow chart RobotControlLib/DIAG_Cont/Pumper/MotorFaultMonitor/MotorMoveMonitor/MotorMoveMonitor ==
  settings: description=chart that monitor motor movement. detects if voltage is given to the mode however not encoder indication that the motor is rotating. this means motor is either stuck (high current) or encoder signal has stopped.
  state moveStart
  state moveRefresh
  state moveFault
    en:
    motorFaultFlag = true;
  (default) -> moveRefresh
  moveRefresh -> moveStart : [moveFlag]/tempDist = motorDist;
  moveStart -> (junction 6) : [after(CONST_ENCOD_TIMER_FAULT, tick) ...
      | || (moveFlag == false)]
  (junction 6) -> moveRefresh [order 2]
  (junction 6) -> moveFault [order 1] : [(moveFlag == true) &&...
      | (motorDist == tempDist)]
  data: tempDist local single; motorDist input; moveFlag input; motorFaultFlag output boolean; CONST_ENCOD_TIMER_FAULT constant uint8 =CONST_ENCOD_TIMER_FAULT
